simulink model "ClosedLoop_Cq"  (R2023b)
settings: Solver=VariableStepAuto  StartTime=0.0  StopTime=10.0  RelTol=1e-3
libraries: cstblocks x3
settings Model: Creator=randolf  LastModifiedBy=randolf

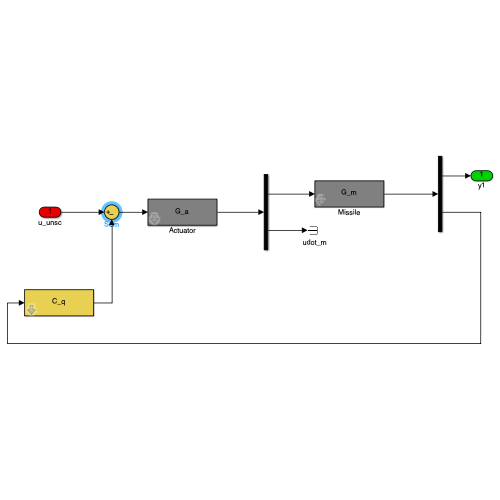
[thumbnail: Simulink's stored preview of the top-level diagram]
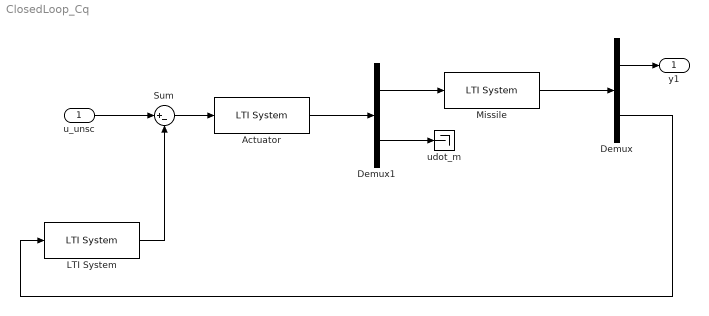
== system ClosedLoop_Cq ==
  u_unsc : Inport
  Actuator : cstblocks/LTI System  sys=G_a  IC=[]  PadeOrder=0
  Demux : Demux  Outputs=2
  Demux1 : Demux  Outputs=2
  LTI System : cstblocks/LTI System  sys=C_q  IC=[]  PadeOrder=0
  Missile : cstblocks/LTI System  sys=G_m  IC=[]  PadeOrder=0
  Sum : Sum  Inputs=|+-
  udot_m : Terminator
  y1 : Outport
  wires:
  Demux/1 -> y1/1
  Demux1/2 -> udot_m/1
  Actuator/1 -> Demux1/1
  Demux/2 -> LTI System/1
  Demux1/1 -> Missile/1
  Missile/1 -> Demux/1
  Sum/1 -> Actuator/1
  u_unsc/1 -> Sum/1
  LTI System/1 -> Sum/2
